simulink model "servo"  (Simulink 8.1)
settings: Solver=ode45  StartTime=0.0  StopTime=10.0  RelTol=1e-3
values from neighbouring files (symbols this model uses):
  J = 0.05    [servo_2_proc.m]    (also in servo_3_proc.m; servo_4_proc.m; servo_proc.m; sys2order_post.m)
  psi = 0.5    [servo_2_proc.m]    (also in servo_3_proc.m; servo_4_proc.m; servo_proc.m; sys2order_post.m)
  R = 10    [servo_2_proc.m]    (also in servo_3_proc.m; servo_4_proc.m; servo_proc.m; sys2order_post.m)
  rho = 2e-4    (= 0.0002)    [servo_2_proc.m]    (also in servo_3_proc.m; servo_4_proc.m; servo_proc.m; sys2order_post.m)
settings Model: Creator=mainster  LastModifiedBy=mainster  BufferReuse=off
settings OptimizationCC: InlineParams=on  BufferReuse=off
settings DebuggingCC: SolverPrmCheckMsg=none  FrameProcessingCompatibilityMsg=error  InitInArrayFormatMsg=none
settings GRTTargetCC: CodeReplacementLibrary=None  CPPClassGenCompliant=on

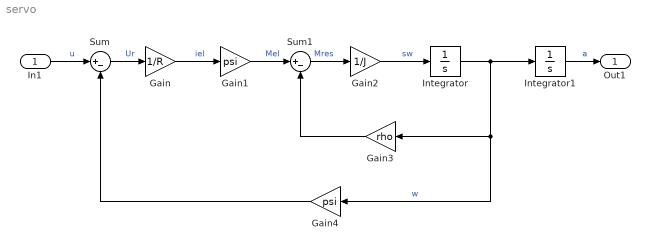
== system servo ==
  In1 : Inport
  Gain : Gain  Gain=1/R
  Gain1 : Gain  Gain=psi
  Gain2 : Gain  Gain=1/J
  Gain3 : Gain  Gain=rho
  Gain4 : Gain  Gain=psi
  Integrator : Integrator
  Integrator1 : Integrator
  Sum : Sum  Inputs=|+-
  Sum1 : Sum  Inputs=|+-
  Out1 : Outport
  wires:
  In1/1 -> Sum/1  "u"
  Sum/1 -> Gain/1  "Ur"
  Gain/1 -> Gain1/1  "iel"
  Gain1/1 -> Sum1/1  "Mel"
  Sum1/1 -> Gain2/1  "Mres"
  Gain2/1 -> Integrator/1  "sw"
  Integrator/1 -> Integrator1/1, Gain3/1, Gain4/1  "w"
  Integrator1/1 -> Out1/1  "a"
  Gain4/1 -> Sum/2
  Gain3/1 -> Sum1/2
